simulink model "Modele_Non_Lineaire_Asservi"  (R2024a)
settings: Solver=VariableStepAuto  StartTime=0.0  StopTime=3  RelTol=1e-3
values from neighbouring files (symbols this model uses):
  den_mot_simu = [R_m*J_eq  (R_m*B_eq+n_g*n_m*k_m*k_t*K_g.^2)]    [Code.m]    (also in Initialisation.m)
  g = 9.81    [Code.m]    (also in Initialisation.m)
  K_int = real((((-1)*den_mot(1)*(Inter^2)) + ((-1)*den_mot(2)*(Inter^1))) / (num_mot(1)))    [Code.m]    (also in Initialisation.m)
  num_mot_simu = [K_g*n_m*n_g*k_t]    [Code.m]    (also in Initialisation.m)
  r_arm = 0.0254    [Code.m]    (also in Initialisation.m)
  Test_Position = 0.06    [Code.m]    (also in Initialisation.m)
  X_den = TF_PD_Bode_Den    [Code.m]    (also in Initialisation.m)
  X_num = TF_PD_Bode_Num    [Code.m]    (also in Initialisation.m)
undefined symbols (not defined in the file or in its folder): L
settings Model: Creator=Mathys  LastModifiedBy=francoisdesautels
settings RTWCC: GPUComputeCapability=3.5

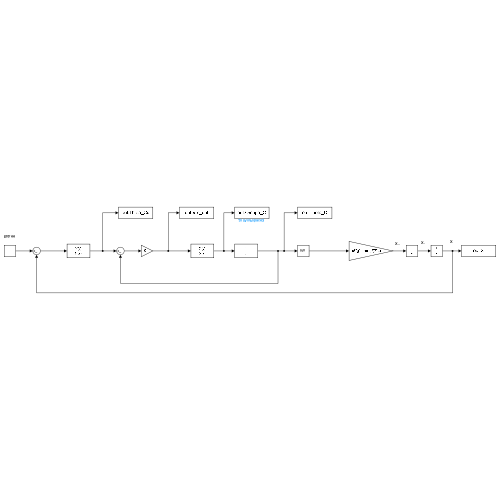
[thumbnail: Simulink's stored preview of the top-level diagram]
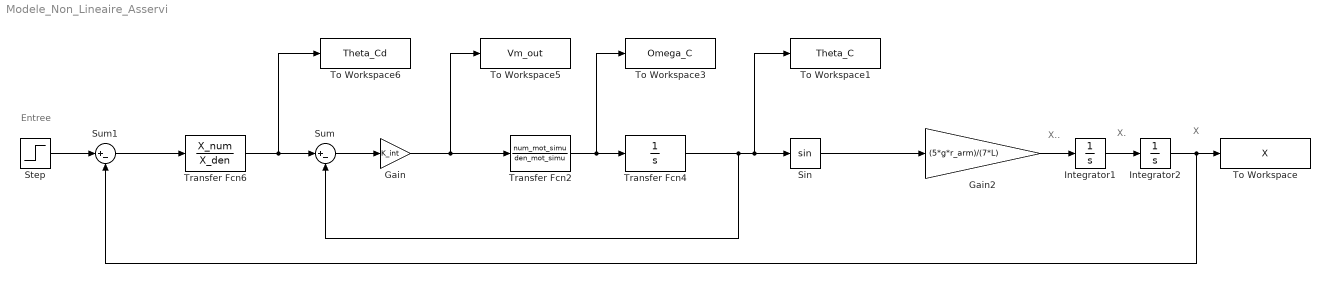
== system Modele_Non_Lineaire_Asservi ==
  note: X
  note: X.
  note: X..
  note: Entree
  Gain : Gain  Gain=K_int
  Gain2 : Gain  Gain=(5*g*r_arm)/(7*L)
  Integrator1 : Integrator
  Integrator2 : Integrator
  Sin : Trigonometry
  Step : Step  After=Test_Position  SampleTime=0
  Sum : Sum  Inputs=|+-
  Sum1 : Sum  Inputs=|+-
  To Workspace : ToWorkspace  VariableName=X  SaveFormat=Timeseries  SampleTime=-1
  To Workspace1 : ToWorkspace  VariableName=Theta_C  SaveFormat=Timeseries  SampleTime=-1
      settings: Save2DSignal=2-D array (concatenate along first dimension)
  To Workspace3 : ToWorkspace  VariableName=Omega_C  SampleTime=-1
  To Workspace5 : ToWorkspace  VariableName=Vm_out  SaveFormat=Timeseries  SampleTime=-1
      settings: Save2DSignal=2-D array (concatenate along first dimension)
  To Workspace6 : ToWorkspace  VariableName=Theta_Cd  SaveFormat=Timeseries  SampleTime=-1
      settings: Save2DSignal=2-D array (concatenate along first dimension)
  Transfer Fcn2 : TransferFcn  Numerator=num_mot_simu  Denominator=den_mot_simu
  Transfer Fcn4 : TransferFcn  Denominator=[1 0]
  Transfer Fcn6 : TransferFcn  Numerator=X_num  Denominator=X_den
  wires:
  Sin/1 -> Gain2/1
  Gain2/1 -> Integrator1/1
  Integrator1/1 -> Integrator2/1
  Integrator2/1 -> Sum1/2, To Workspace/1
  Transfer Fcn2/1 -> To Workspace3/1, Transfer Fcn4/1
  Sum/1 -> Gain/1
  Transfer Fcn4/1 -> To Workspace1/1, Sin/1, Sum/2
  Step/1 -> Sum1/1
  Sum1/1 -> Transfer Fcn6/1
  Transfer Fcn6/1 -> To Workspace6/1, Sum/1
  Gain/1 -> To Workspace5/1, Transfer Fcn2/1
